simulink model "Dc_Motor_Position_Crtl_tuning"  (R2020b)
settings: Solver=VariableStepAuto  StartTime=0.0  StopTime=10.0  RelTol=1e-3
values from neighbouring files (symbols this model uses):
  b = 3.5077E-6    (= 3.5077e-06)    [dc_motor_position_crtl.m]    (also in dc_motor_position_crtl_tuning.m)
  J = 3.2284E-6    (= 3.2284e-06)    [dc_motor_position_crtl.m]    (also in dc_motor_position_crtl_tuning.m)
  Kb = 0.0274    [dc_motor_position_crtl.m]    (also in dc_motor_position_crtl_tuning.m)
  Kd = 0    [dc_motor_position_crtl_tuning.m]
  Ki = 0    [dc_motor_position_crtl_tuning.m]
  Kp = 100    [dc_motor_position_crtl_tuning.m]
  Kt = 0.0274    [dc_motor_position_crtl.m]    (also in dc_motor_position_crtl_tuning.m)
  L = 2.75E-6    (= 2.75e-06)    [dc_motor_position_crtl.m]    (also in dc_motor_position_crtl_tuning.m)
  R = 4    [dc_motor_position_crtl.m]    (also in dc_motor_position_crtl_tuning.m)
  V = 1    [dc_motor_position_crtl.m]    (also in dc_motor_position_crtl_tuning.m)
libraries: pid_lib x1
settings Model: Creator=Raihan mahmud  LastModifiedBy=Raihan mahmud

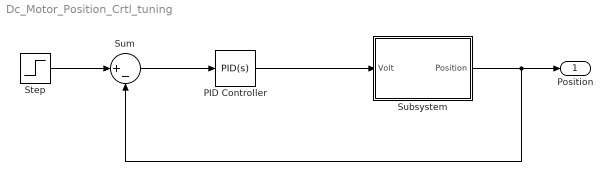
== system Dc_Motor_Position_Crtl_tuning ==
  PID Controller : pid_lib/PID Controller  Controller=PID  Form=Parallel  TimeDomain=Continuous-time  UseExternalTs=off  SampleTime=-1  IntegratorMethod=Forward Euler  FilterMethod=Forward Euler  ControllerParametersSource=internal  P=Kp  I=Ki  D=Kd  UseFilter=on  N=100  TunerSelectOption=Transfer Function Based (PID Tuner App)  InitialConditionSource=internal  InitialConditionForIntegrator=0  InitialConditionForFilter=0  DifferentiatorICPrevScaledInput=0  ExternalReset=none  TrackingMode=off  Kt=1  LimitOutput=off  SatLimitsSource=internal  UpperSaturationLimit=inf  LowerSaturationLimit=-inf  LinearizeAsGain=on  AntiWindupMode=none  Kb=1  POutMin=[]  POutMax=[]  IOutMin=[]  IOutMax=[]  DOutMin=[]  DOutMax=[]  NOutMin=[]  NOutMax=[]  SumOutMin=[]  SumOutMax=[]  SaturationOutMin=[]  SaturationOutMax=[]  PParamMin=[]  PParamMax=[]  IParamMin=[]  IParamMax=[]  DParamMin=[]  DParamMax=[]  NParamMin=[]  NParamMax=[]  KbParamMin=[]  KbParamMax=[]  KtParamMin=[]  KtParamMax=[]  KbOutMin=[]  KbOutMax=[]  KtOutMin=[]  KtOutMax=[]  IntegratorOutMin=[]  IntegratorOutMax=[]  FilterOutMin=[]  FilterOutMax=[]  SumI1OutMin=[]  SumI1OutMax=[]  SumI2OutMin=[]  SumI2OutMax=[]  SumI3OutMin=[]  SumI3OutMax=[]  SumI4OutMin=[]  SumI4OutMax=[]  SumDOutMin=[]  SumDOutMax=[]  DifferentiatorOutMin=[]  DifferentiatorOutMax=[]  FilterDiffOutCoefMin=[]  FilterDiffOutCoefMax=[]  ReciprocalOutMin=[]  ReciprocalOutMax=[]  SumDenOutMin=[]  SumDenOutMax=[]  SumNumOutMin=[]  SumNumOutMax=[]  DivideOutMin=[]  DivideOutMax=[]  UdiffTsProdOutMin=[]  UdiffTsProdOutMax=[]  NTsProdOutMin=[]  NTsProdOutMax=[]  UintegralTsProdOutMin=[]  UintegralTsProdOutMax=[]  UngainTsProdOutMin=[]  UngainTsProdOutMax=[]  IntegratorContinuousStateAttributes=''  IntegratorStateMustResolveToSignalObject=off  IntegratorRTWStateStorageClass=Auto  FilterContinuousStateAttributes=''  FilterStateMustResolveToSignalObject=off  FilterRTWStateStorageClass=Auto  ParallelPVariant=InternalParameters  IdealPVariant=Disabled  IVariant=InternalParameters  DVariant=InternalParameters  IntegratorVariant=Continuous  SatVariant=Disabled  AWVariant=Passthrough  PCopyVariant=Disabled  TRVariant=Disabled  FdbkBlocksVariant=Forward  IdealPFdbkVariant=Disabled  SatFdbkVariant=Disabled  DerivativeFilterVariant=ContFilter  NVariant=InternalParameters  NCopyVariant=Disabled  FilterICVariant=InternalICsFilter  IntegratorICVariant=InternalICs  ExternalResetVariant=Disabled  TRSumVariant=Passthrough  SumFdbkVariant=Disabled  SumVariant=Sum_PID  TsampFilterVariant=InternalTs  TsampNgainVariant=Passthrough  TsampIntegralVariant=Passthrough  ExternalSaturationOutDataTypeStr=Inherit: Same as second input
  Step : Step  Time=V  SampleTime=0
  Subsystem : Subsystem
  Sum : Sum  Inputs=|+-
  Position : Outport
  wires:
  Sum/1 -> PID Controller/1
  Subsystem/1(Position) -> Sum/2, Position/1
  PID Controller/1 -> Subsystem/1(Volt)
  Step/1 -> Sum/1

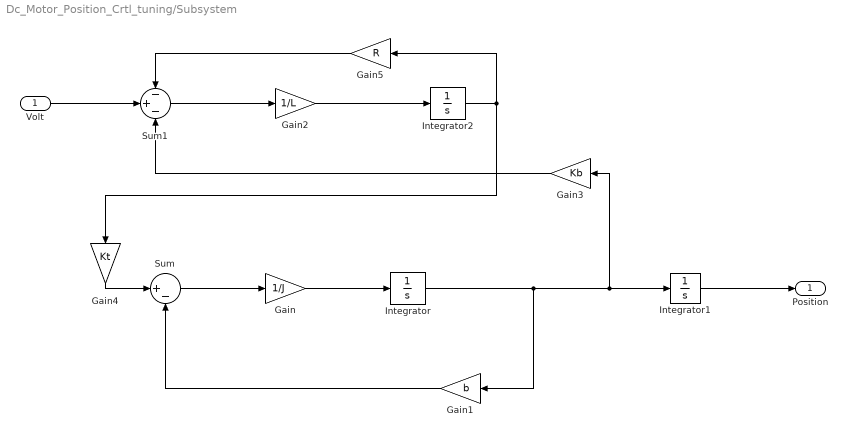
== system Dc_Motor_Position_Crtl_tuning/Subsystem ==
  Volt : Inport
  Gain : Gain  Gain=1/J
  Gain1 : Gain  Gain=b
  Gain2 : Gain  Gain=1/L
  Gain3 : Gain  Gain=Kb
  Gain4 : Gain  Gain=Kt
  Gain5 : Gain  Gain=R
  Integrator : Integrator
  Integrator1 : Integrator
  Integrator2 : Integrator
  Sum : Sum  Inputs=|+-
  Sum1 : Sum  Inputs=-+-
  Position : Outport
  wires:
  Gain3/1 -> Sum1/3
  Integrator/1 -> Gain3/1, Integrator1/1, Gain1/1
  Integrator2/1 -> Gain5/1, Gain4/1
  Gain1/1 -> Sum/2
  Sum/1 -> Gain/1
  Sum1/1 -> Gain2/1
  Gain5/1 -> Sum1/1
  Gain/1 -> Integrator/1
  Gain2/1 -> Integrator2/1
  Gain4/1 -> Sum/1
  Volt/1 -> Sum1/2
  Integrator1/1 -> Position/1
